simulink model "model_affc"  (R2016b)
settings: Solver=FixedStepDiscrete  StartTime=0.0  StopTime=inf  FixedStep=sampleTime  RelTol=1e-3
PostLoadFcn:
  | model_affc_parameters;
InitFcn:
  | model_affc_parameters;
StartFcn:
  | model_affc_parameters;
values from neighbouring files (symbols this model uses):
  Lb = 0.07    [model_affc_parameters.m]    (also in parameters_sysid.m; parameters_sysid_admittance.m)
  Lf = 0.238    [model_affc_parameters.m]    (also in parameters_sysid.m; parameters_sysid_admittance.m)
  Lu = 0.153    [model_affc_parameters.m]    (also in parameters_sysid.m; parameters_sysid_admittance.m)
  sampleTime = 0.001    [model_affc_parameters.m]    (also in parameters_sysid.m; parameters_sysid_admittance.m)
undefined symbols (not defined in the file or in its folder): FM1
libraries: simulink x14, LibraryFM x14
(part 1 of 2)
settings Model: SimulationMode=external  Creator=niekbeckers  LastModifiedBy=Labuser
settings DataIOCC: LimitDataPoints=on  SaveFormat=Array
settings OptimizationCC: BlockReduction=off  BooleanDataType=off  LocalBlockOutputs=off  LifeSpan=inf
settings DebuggingCC: SaveWithParameterizedLinksMsg=none  UnderspecifiedInitializationDetection=Classic  MergeDetectMultiDrivingBlocksExec=none  SignalResolutionControl=TryResolveAllWithWarning  SFUnexpectedBacktrackingDiag=warning  SFNoUnconditionalDefaultTransitionDiag=warning  SFExecutionAtInitializationDiag=none
settings HardwareCC: ProdBitPerPointer=32  ProdBitPerSizeT=32  ProdBitPerPtrDiffT=32  ProdLargestAtomicFloat=None  ProdIntDivRoundTo=Undefined  ProdEndianess=Unspecified  ProdWordSize=32  ProdHWDeviceType=32-bit Generic  TargetBitPerPointer=64  TargetBitPerSizeT=64  TargetBitPerPtrDiffT=64  TargetLongLongMode=on  TargetIntDivRoundTo=Zero  TargetEndianess=LittleEndian  TargetWordSize=64  TargetHWDeviceType=MATLAB Host  ProdEqTarget=off
settings ModelReferenceCC: PropagateSignalLabelsOutOfModel=off
settings RTWCC: SystemTargetFile=TwinCAT.tlc  GenCodeOnly=on  MakeCommand=make_tct  TemplateMakefile=tct_msbuild.tmf  Description=TwinCAT Target  GenerateReport=on  TargetLang=C++
settings STFCustomTargetCC: CompOptLevelCompliant=on  GeneratePreprocessorConditionals=Disable all  MATLABClassNameForMDSCustomization=Simulink.SoftwareTarget.TargetSpecificTriggerConfigurationBase  SystemTargetFile=TwinCAT.tlc
settings ConfigComp: CovMetricSettings=dw  CovHtmlReporting=on  CovSaveCumulativeToWorkspaceVar=on  CovSaveSingleToWorkspaceVar=on  CovExternalEMLEnable=off  CovSFcnEnable=off

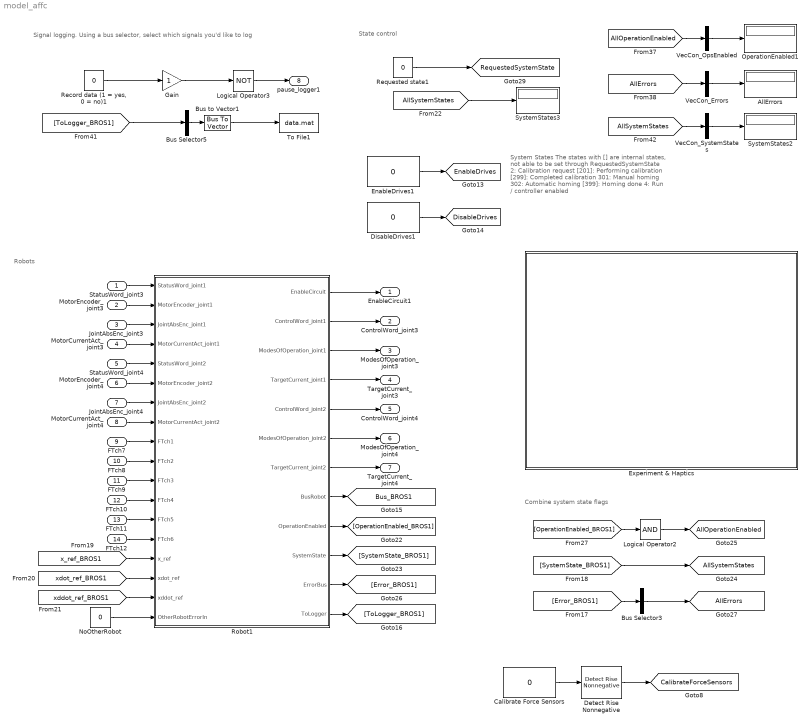
== system model_affc ==
  note: Signal logging.
      | Using a bus selector, select which signals you'd like to log
  note: System States
      | The states with [] are internal states, not able to be set through RequestedSystemState
      | 2: Calibration request
      | [201]: Performing calibration
      | [299]: Completed calibration
      | 301: Manual homing
      | 302: Automatic homing
      | [399]: Homing done
      | 4: Run / controller enabled
  note: State control
  note: Combine system state flags
  note: Robots
  StatusWord_joint3 : Inport  OutDataTypeStr=uint16  PortDimensions=1
  MotorEncoder_joint3 : Inport  Port=2  OutDataTypeStr=int32  PortDimensions=1
  JointAbsEnc_joint3 : Inport  Port=3  OutDataTypeStr=int32  PortDimensions=1
  MotorCurrentAct_joint3 : Inport  Port=4  OutDataTypeStr=int16  PortDimensions=1
  StatusWord_joint4 : Inport  Port=5  OutDataTypeStr=uint16  PortDimensions=1
  MotorEncoder_joint4 : Inport  Port=6  OutDataTypeStr=int32  PortDimensions=1
  JointAbsEnc_joint4 : Inport  Port=7  OutDataTypeStr=int32  PortDimensions=1
  MotorCurrentAct_joint4 : Inport  Port=8  OutDataTypeStr=int16  PortDimensions=1
  FTch7 : Inport  Port=9  OutDataTypeStr=single  PortDimensions=1
  FTch8 : Inport  Port=10  OutDataTypeStr=single  PortDimensions=1
  FTch9 : Inport  Port=11  OutDataTypeStr=single  PortDimensions=1
  FTch10 : Inport  Port=12  OutDataTypeStr=single  PortDimensions=1
  FTch11 : Inport  Port=13  OutDataTypeStr=single  PortDimensions=1
  FTch12 : Inport  Port=14  OutDataTypeStr=single  PortDimensions=1
  AllErrors : Display
  Bus Selector3 : BusSelector  OutputSignals=ErrorCodeLatched  OutputAsBus=on
  Bus Selector5 : BusSelector  OutputSignals=SystemState,qJointSpace.q,qJointSpace.qdot,xOpSpace.x,xOpSpace.xdot,Controller_ToLogger.q_ref,Controller_ToLogger.qdot_ref,Controller_ToLogger.qddot_ref,Controller_ToLogger.p,Controller_ToLogger.tau_affc,BusFTSensor.ForcesOpSpace,ToEtherCAT_ToLogger_Actuator1.DriveError,ToEtherCAT_ToLogger_Actuator2.DriveError  OutputAsBus=on
  Bus to Vector1 : BusToVector
  Calibrate Force Sensors : Constant  Value=0
      settings: OpenFcn=set_param(gcb,'Value','1');tname = ['toggletimer_' gcb];delete(timerfind('name',tname));t = timer('timerfcn', ['set_param(''',gcb,''',''Value'',''0'')'],'executionmode','singleshot','startdelay',1,'name',tname);start(t);
      mask Display: fprintf('PushToTrigger\n%s',get_param(gcb,'value'))
  Detect Rise Nonnegative : simulink/Logic and Bit Operations/Detect Rise Nonnegative  vinit=0  OutDataTypeStr=boolean
  DisableDrives1 : Constant  Value=0
      settings: OpenFcn=set_param(gcb,'Value','1');tname = ['toggletimer_' gcb];delete(timerfind('name',tname));t = timer('timerfcn', ['set_param(''',gcb,''',''Value'',''0'')'],'executionmode','singleshot','startdelay',1,'name',tname);start(t);
      mask Display: fprintf('PushToTrigger\n%s',get_param(gcb,'value'))
  EnableDrives1 : Constant  Value=0
      settings: OpenFcn=set_param(gcb,'Value','1');tname = ['toggletimer_' gcb];delete(timerfind('name',tname));t = timer('timerfcn', ['set_param(''',gcb,''',''Value'',''0'')'],'executionmode','singleshot','startdelay',1,'name',tname);start(t);
      mask Display: fprintf('PushToTrigger\n%s',get_param(gcb,'value'))
  Experiment & Haptics : Subsystem
  Gain : Gain
  Logical Operator2 : Logic  Inputs=1  AllPortsSameDT=off  OutDataTypeStr=boolean
  Logical Operator3 : Logic  Operator=NOT  Inputs=1  AllPortsSameDT=off  OutDataTypeStr=boolean
  NoOtherRobot : Constant  Value=0
  OperationEnabled1 : Display
  "Record data (1 = yes, 0 = no)1" : Constant  Value=0
  Requested state1 : Constant  Value=0
  Robot1 : Subsystem  mask{RobotStruct=FM1}
      mask prompts: RobotStruct "Robot struct (data)"
  SystemStates2 : Display
  SystemStates3 : Display
  To File1 : ToFile  Filename=data.mat  MatrixName=data
  VecCon_Errors : Concatenate  NumInputs=1
  VecCon_OpsEnabled : Concatenate  NumInputs=1
  VecCon_SystemStates : Concatenate  NumInputs=1
  EnableCircuit1 : Outport  OutDataTypeStr=boolean  PortDimensions=1
  ControlWord_joint3 : Outport  Port=2  OutDataTypeStr=uint16  PortDimensions=1
  ModesOfOperation_joint3 : Outport  Port=3  OutDataTypeStr=int8  PortDimensions=1
  TargetCurrent_joint3 : Outport  Port=4  OutDataTypeStr=int16  PortDimensions=1
  ControlWord_joint4 : Outport  Port=5  OutDataTypeStr=uint16  PortDimensions=1
  ModesOfOperation_joint4 : Outport  Port=6  OutDataTypeStr=int8  PortDimensions=1
  TargetCurrent_joint4 : Outport  Port=7  OutDataTypeStr=int16  PortDimensions=1
  pause_logger1 : Outport  Port=8  OutDataTypeStr=boolean  PortDimensions=1
  tag scope: AllErrors=global, AllOperationEnabled=global, AllSystemStates=global, Bus_BROS1=global, CalibrateForceSensors=global, DisableDrives=global, EnableDrives=global, RequestedSystemState=global
  wires:
  DisableDrives1/1 -> [DisableDrives]
  EnableDrives1/1 -> [EnableDrives]
  Robot1/9(OperationEnabled) -> [OperationEnabled_BROS1]
  [AllOperationEnabled] -> VecCon_OpsEnabled/1
  Robot1/10(SystemState) -> [SystemState_BROS1]
  [SystemState_BROS1] -> [AllSystemStates]
  Logical Operator2/1 -> [AllOperationEnabled]
  [OperationEnabled_BROS1] -> Logical Operator2/1
  Robot1/11(ErrorBus) -> [Error_BROS1]
  [Error_BROS1] -> Bus Selector3/1
  [AllErrors] -> VecCon_Errors/1
  [x_ref_BROS1] -> Robot1/15(x_ref)
  [xdot_ref_BROS1] -> Robot1/16(xdot_ref)
  [xddot_ref_BROS1] -> Robot1/17(xddot_ref)
  Requested state1/1 -> [RequestedSystemState]
  Robot1/8(BusRobot) -> [Bus_BROS1]
  StatusWord_joint3/1 -> Robot1/1(StatusWord_joint1)
  MotorEncoder_joint3/1 -> Robot1/2(MotorEncoder_joint1)
  JointAbsEnc_joint3/1 -> Robot1/3(JointAbsEnc_joint1)
  MotorCurrentAct_joint3/1 -> Robot1/4(MotorCurrentAct_joint1)
  StatusWord_joint4/1 -> Robot1/5(StatusWord_joint2)
  MotorEncoder_joint4/1 -> Robot1/6(MotorEncoder_joint2)
  JointAbsEnc_joint4/1 -> Robot1/7(JointAbsEnc_joint2)
  MotorCurrentAct_joint4/1 -> Robot1/8(MotorCurrentAct_joint2)
  FTch7/1 -> Robot1/9(FTch1)
  FTch8/1 -> Robot1/10(FTch2)
  FTch9/1 -> Robot1/11(FTch3)
  FTch10/1 -> Robot1/12(FTch4)
  FTch11/1 -> Robot1/13(FTch5)
  FTch12/1 -> Robot1/14(FTch6)
  Robot1/2(ControlWord_joint1) -> ControlWord_joint3/1
  Robot1/3(ModesOfOperation_joint1) -> ModesOfOperation_joint3/1
  Robot1/4(TargetCurrent_joint1) -> TargetCurrent_joint3/1
  Robot1/7(TargetCurrent_joint2) -> TargetCurrent_joint4/1
  Robot1/6(ModesOfOperation_joint2) -> ModesOfOperation_joint4/1
  Robot1/5(ControlWord_joint2) -> ControlWord_joint4/1
  Robot1/12(ToLogger) -> [ToLogger_BROS1]
  [ToLogger_BROS1] -> Bus Selector5/1
  [AllSystemStates] -> SystemStates3/1
  Logical Operator3/1 -> pause_logger1/1
  Bus Selector5/1 -> Bus to Vector1/1
  Bus Selector3/1 -> [AllErrors]
  Bus to Vector1/1 -> To File1/1
  Robot1/1(EnableCircuit) -> EnableCircuit1/1
  NoOtherRobot/1 -> Robot1/18(OtherRobotErrorIn)
  VecCon_Errors/1 -> AllErrors/1
  [AllSystemStates] -> VecCon_SystemStates/1
  VecCon_SystemStates/1 -> SystemStates2/1
  VecCon_OpsEnabled/1 -> OperationEnabled1/1
  "Record data (1 = yes, 0 = no)1"/1 -> Gain/1
  Calibrate Force Sensors/1 -> Detect Rise Nonnegative/1
  Detect Rise Nonnegative/1 -> [CalibrateForceSensors]
  Gain/1 -> Logical Operator3/1

== system model_affc/Experiment & Haptics ==
  note: Only run trajectory if all systems are in state 4 (run)
  Add : Sum
  "Check state " : simulink/Logic and Bit Operations/Compare To Constant  relop===  const=4  OutDataTypeStr=boolean
  Constant : Constant  Value=FM1.HomeLocationOpSpace
  Hypotrochoid trajectory for AFFC : Subsystem
  Logical Operator : Logic  Inputs=1  AllPortsSameDT=off  OutDataTypeStr=boolean
  Terminator1 : Terminator
  tag scope: x_ref_BROS1=global, xddot_ref_BROS1=global, xdot_ref_BROS1=global
  wires:
  [Bus_BROS1] -> Terminator1/1
  Constant/1 -> Add/1
  Hypotrochoid trajectory for AFFC/1(dx_ref) -> Add/2
  Add/1 -> [x_ref_BROS1]
  Hypotrochoid trajectory for AFFC/2(dxdot_ref) -> [xdot_ref_BROS1]
  Hypotrochoid trajectory for AFFC/3(dxddot_ref) -> [xddot_ref_BROS1]
  [AllSystemStates] -> "Check state "/1
  "Check state "/1 -> Logical Operator/1
  Logical Operator/1 -> Hypotrochoid trajectory for AFFC/Enable

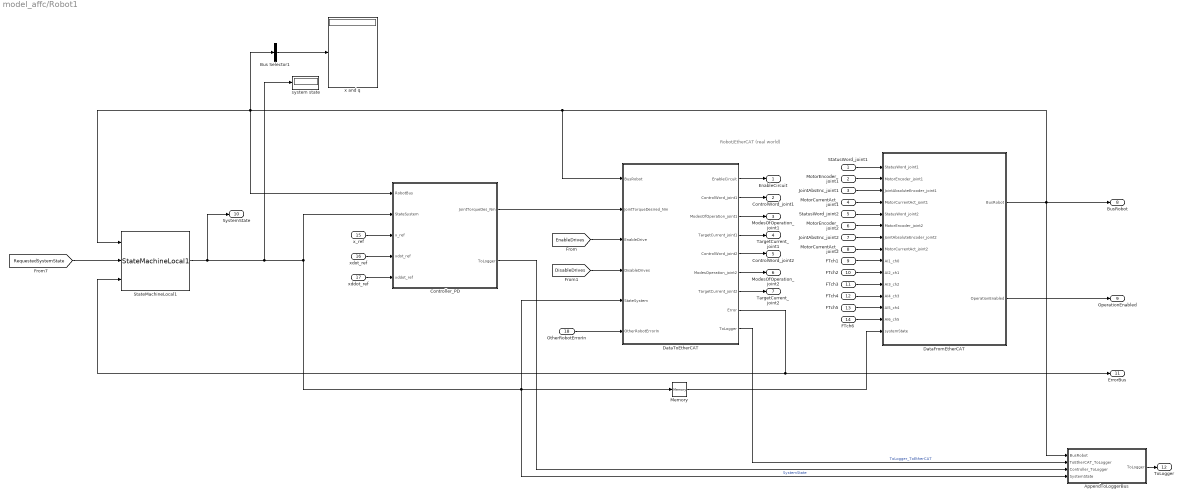
== system model_affc/Robot1 ==
  note: Robot/EtherCAT (real world)
  StatusWord_joint1 : Inport
  MotorEncoder_joint1 : Inport  Port=2
  JointAbsEnc_joint1 : Inport  Port=3
  MotorCurrentAct_joint1 : Inport  Port=4
  StatusWord_joint2 : Inport  Port=5
  MotorEncoder_joint2 : Inport  Port=6
  JointAbsEnc_joint2 : Inport  Port=7
  MotorCurrentAct_joint2 : Inport  Port=8
  FTch1 : Inport  Port=9
  FTch2 : Inport  Port=10
  FTch3 : Inport  Port=11
  FTch4 : Inport  Port=12
  FTch5 : Inport  Port=13
  FTch6 : Inport  Port=14
  x_ref : Inport  Port=15
  xdot_ref : Inport  Port=16
  xddot_ref : Inport  Port=17
  OtherRobotErrorIn : Inport  Port=18
  AppendToLoggerBus : Subsystem
  Bus Selector1 : BusSelector  OutputSignals=qJointSpace.q,qJointSpace.qdot,xOpSpace.x,BusActuators.BusActuator1.JointPosition_AbsEnc_rad,BusActuators.BusActuator2.JointPosition_AbsEnc_rad  OutputAsBus=on
  Controller_PD : Subsystem
  DataFromEtherCAT : Subsystem
  DataToEtherCAT : Subsystem
  Memory : Memory
  StateMachineLocal1 : LibraryFM/StateMachineLocal1
  system state : Display
  x and q : Display
  EnableCircuit : Outport
  ControlWord_joint1 : Outport  Port=2
  ModesOfOperation_joint1 : Outport  Port=3
  TargetCurrent_joint1 : Outport  Port=4
  ControlWord_joint2 : Outport  Port=5
  ModesOfOperation_joint2 : Outport  Port=6
  TargetCurrent_joint2 : Outport  Port=7
  BusRobot : Outport  Port=8
  OperationEnabled : Outport  Port=9
  SystemState : Outport  Port=10
  ErrorBus : Outport  Port=11
  ToLogger : Outport  Port=12
  wires:
  xddot_ref/1 -> Controller_PD/5(xddot_ref)
  xdot_ref/1 -> Controller_PD/4(xdot_ref)
  x_ref/1 -> Controller_PD/3(x_ref)
  DataToEtherCAT/7(TargetCurrent_joint2) -> TargetCurrent_joint2/1
  FTch2/1 -> DataFromEtherCAT/10(AI2_ch1)
  MotorCurrentAct_joint1/1 -> DataFromEtherCAT/4(MotorCurrentAct_joint1)
  MotorEncoder_joint2/1 -> DataFromEtherCAT/6(MotorEncoder_joint2)
  JointAbsEnc_joint1/1 -> DataFromEtherCAT/3(JointAbsoluteEncoder_joint1)
  DataToEtherCAT/3(ModesOfOperation_joint1) -> ModesOfOperation_joint1/1
  DataToEtherCAT/1(EnableCircuit) -> EnableCircuit/1
  FTch1/1 -> DataFromEtherCAT/9(AI1_ch0)
  StateMachineLocal1/1 -> system state/1, Controller_PD/2(StateSystem), DataToEtherCAT/5(StateSystem), Memory/1, AppendToLoggerBus/4(SystemState), SystemState/1  "SystemState"
  DataToEtherCAT/2(ControlWord_joint1) -> ControlWord_joint1/1
  DataToEtherCAT/8(Error) -> StateMachineLocal1/3, ErrorBus/1
  DataFromEtherCAT/1(BusRobot) -> AppendToLoggerBus/1(BusRobot), Controller_PD/1(RobotBus), StateMachineLocal1/1, Bus Selector1/1, DataToEtherCAT/1(BusRobot), BusRobot/1
  [RequestedSystemState] -> StateMachineLocal1/2
  Controller_PD/1(JointTorqueDes_Nm) -> DataToEtherCAT/2(JointTorqueDesired_Nm)
  [DisableDrives] -> DataToEtherCAT/4(DisableDrives)
  [EnableDrives] -> DataToEtherCAT/3(EnableDrive)
  MotorCurrentAct_joint2/1 -> DataFromEtherCAT/8(MotorCurrentAct_joint2)
  DataToEtherCAT/4(TargetCurrent_joint1) -> TargetCurrent_joint1/1
  FTch5/1 -> DataFromEtherCAT/13(AI5_ch4)
  JointAbsEnc_joint2/1 -> DataFromEtherCAT/7("JointAbsoluteEncoder_joint2 ")
  MotorEncoder_joint1/1 -> DataFromEtherCAT/2(MotorEncoder_joint1)
  DataToEtherCAT/5(ControlWord_joint2) -> ControlWord_joint2/1
  DataToEtherCAT/6(ModesOperation_joint2) -> ModesOfOperation_joint2/1
  StatusWord_joint1/1 -> DataFromEtherCAT/1(StatusWord_joint1)
  StatusWord_joint2/1 -> DataFromEtherCAT/5(StatusWord_joint2)
  FTch6/1 -> DataFromEtherCAT/14(AI6_ch5)
  FTch4/1 -> DataFromEtherCAT/12(AI4_ch3)
  FTch3/1 -> DataFromEtherCAT/11(AI3_ch2)
  DataFromEtherCAT/2(OperationEnabled) -> OperationEnabled/1
  Bus Selector1/1 -> x and q/1
  Controller_PD/2(ToLogger) -> AppendToLoggerBus/3(Controller_ToLogger)
  DataToEtherCAT/9(ToLogger) -> AppendToLoggerBus/2(ToEtherCAT_ToLogger)  "ToLogger_ToEtherCAT"
  AppendToLoggerBus/1(ToLogger) -> ToLogger/1
  Memory/1 -> DataFromEtherCAT/15(systemState)
  OtherRobotErrorIn/1 -> DataToEtherCAT/6(OtherRobotErrorIn)

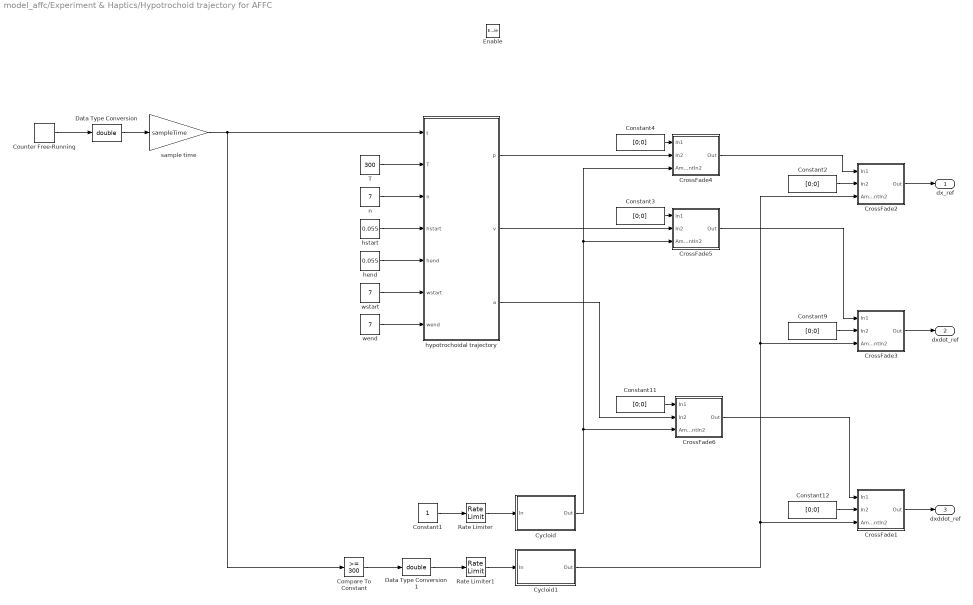
== system model_affc/Experiment & Haptics/Hypotrochoid trajectory for AFFC ==
  Enable : EnablePort  StatesWhenEnabling=reset
  Compare To Constant : simulink/Logic and Bit Operations/Compare To Constant  relop=>=  const=300  OutDataTypeStr=boolean
  Constant1 : Constant
  Constant{2..4,9,11..12} (6 alike) : Constant  Value=[0;0]
  Counter Free-Running : simulink/Sources/Counter Free-Running  NumBits=32  tsamp=-1
  CrossFade1 : Subsystem  AncestorBlock=VariousBlocksLibrary/Various/CrossFade
  CrossFade2 : Subsystem  AncestorBlock=VariousBlocksLibrary/Various/CrossFade
  CrossFade3 : Subsystem  AncestorBlock=VariousBlocksLibrary/Various/CrossFade
  CrossFade4 : Subsystem
  CrossFade5 : Subsystem  AncestorBlock=VariousBlocksLibrary/Various/CrossFade
  CrossFade6 : Subsystem  AncestorBlock=VariousBlocksLibrary/Various/CrossFade
  Cycloid : Subsystem  AncestorBlock=VariousBlocksLibrary/Various/Cycloid
  Cycloid1 : Subsystem  AncestorBlock=VariousBlocksLibrary/Various/Cycloid
  Data Type Conversion : DataTypeConversion  OutDataTypeStr=double
  Data Type Conversion1 : DataTypeConversion  OutDataTypeStr=double
  Rate Limiter : RateLimiter  RisingSlewLimit=0.25  FallingSlewLimit=-0.15  SampleTimeMode=inherited
  Rate Limiter1 : RateLimiter  RisingSlewLimit=0.2  FallingSlewLimit=-0.2  SampleTimeMode=inherited
  T : Constant  Value=300
  hend : Constant  Value=0.055
  hstart : Constant  Value=0.055
  hypotrochoidal trajectory : MATLAB Function  TreatAsAtomicUnit=on
  n : Constant  Value=7
  sample time : Gain  Gain=sampleTime
  wend : Constant  Value=7
  wstart : Constant  Value=7
  dx_ref : Outport  InitialOutput=[0;0]
  dxdot_ref : Outport  Port=2  InitialOutput=[0;0]
  dxddot_ref : Outport  Port=3  InitialOutput=[0;0]
  wires:
  Data Type Conversion1/1 -> Rate Limiter1/1
  hypotrochoidal trajectory/1(p) -> CrossFade4/2(In2)
  CrossFade1/1(Out) -> dxddot_ref/1
  Constant11/1 -> CrossFade6/1(In1)
  Constant12/1 -> CrossFade1/2(In2)
  CrossFade6/1(Out) -> CrossFade1/1(In1)
  Constant9/1 -> CrossFade3/2(In2)
  CrossFade5/1(Out) -> CrossFade3/1(In1)
  CrossFade3/1(Out) -> dxdot_ref/1
  Cycloid1/1(Out) -> CrossFade1/3(AmountIn2), CrossFade2/3(AmountIn2), CrossFade3/3(AmountIn2)
  Rate Limiter1/1 -> Cycloid1/1(In)
  Compare To Constant/1 -> Data Type Conversion1/1
  CrossFade4/1(Out) -> CrossFade2/1(In1)
  CrossFade2/1(Out) -> dx_ref/1
  Rate Limiter/1 -> Cycloid/1(In)
  Constant1/1 -> Rate Limiter/1
  Cycloid/1(Out) -> CrossFade6/3(AmountIn2), CrossFade5/3(AmountIn2), CrossFade4/3(AmountIn2)
  hypotrochoidal trajectory/2(v) -> CrossFade5/2(In2)
  hypotrochoidal trajectory/3(a) -> CrossFade6/2(In2)
  sample time/1 -> Compare To Constant/1, hypotrochoidal trajectory/1(t)
  Constant2/1 -> CrossFade2/2(In2)
  Data Type Conversion/1 -> sample time/1
  wstart/1 -> hypotrochoidal trajectory/6(wstart)
  wend/1 -> hypotrochoidal trajectory/7(wend)
  hstart/1 -> hypotrochoidal trajectory/4(hstart)
  hend/1 -> hypotrochoidal trajectory/5(hend)
  n/1 -> hypotrochoidal trajectory/3(n)
  T/1 -> hypotrochoidal trajectory/2(T)
  Counter Free-Running/1 -> Data Type Conversion/1
  Constant3/1 -> CrossFade5/1(In1)
  Constant4/1 -> CrossFade4/1(In1)

== system model_affc/Robot1/AppendToLoggerBus ==
  BusRobot : Inport
  ToEtherCAT_ToLogger : Inport  Port=2
  Controller_ToLogger : Inport  Port=3
  SystemState : Inport  Port=4
  Bus Creator : BusCreator  Inputs=8
  Bus Selector : BusSelector  OutputSignals=xOpSpace,qJointSpace,BusFTSensor,BusActuators
  Bus Selector1 : BusSelector  OutputSignals=ToEtherCAT_ToLogger_Actuator1,ToEtherCAT_ToLogger_Actuator2
  ToLogger : Outport
  wires:
  Bus Creator/1 -> ToLogger/1  "LoggerBus"
  Bus Selector/4 -> Bus Creator/4  "<BusActuators>"
  Bus Selector/1 -> Bus Creator/1  "<xOpSpace>"
  Bus Selector/3 -> Bus Creator/3  "<BusFTSensor>"
  Bus Selector/2 -> Bus Creator/2  "<qJointSpace>"
  BusRobot/1 -> Bus Selector/1
  ToEtherCAT_ToLogger/1 -> Bus Selector1/1
  Bus Selector1/1 -> Bus Creator/5  "<ToEtherCAT_ToLogger_Actuator1>"
  Bus Selector1/2 -> Bus Creator/6  "<ToEtherCAT_ToLogger_Actuator2>"
  Controller_ToLogger/1 -> Bus Creator/7
  SystemState/1 -> Bus Creator/8  "SystemState"

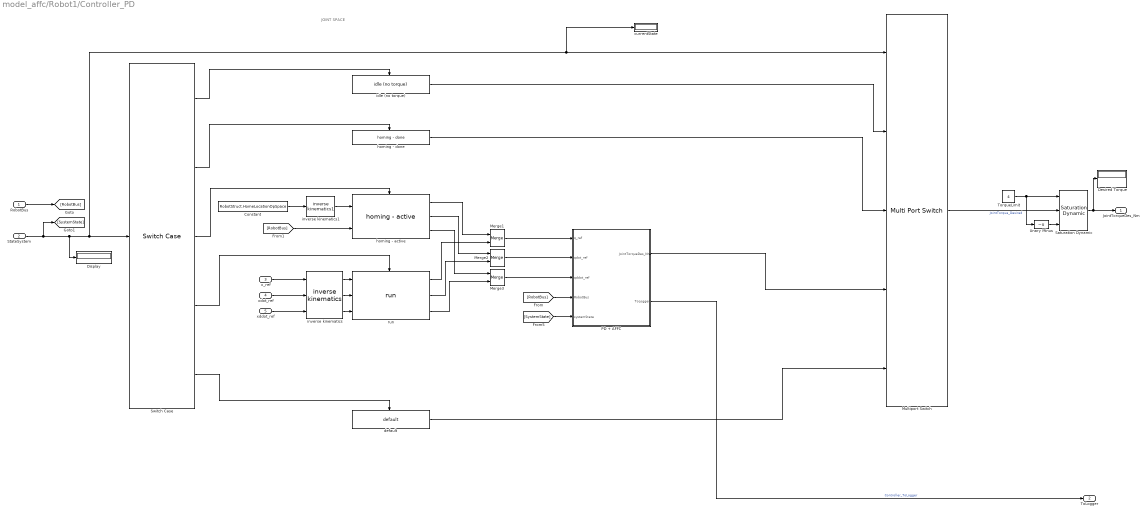
== system model_affc/Robot1/Controller_PD ==
  note: JOINT SPACE
  RobotBus : Inport
  StateSystem : Inport  Port=2
  x_ref : Inport  Port=3
  xdot_ref : Inport  Port=4
  xddot_ref : Inport  Port=5
  Constant : Constant  Value=RobotStruct.HomeLocationOpSpace
  Desired Torque : Display
  Display : Display
  Merge1 : Merge  InitialOutput=[0;0]
  Merge2 : Merge  InitialOutput=[0;0]
  Merge3 : Merge  InitialOutput=[0;0]
  Multiport Switch : MultiPortSwitch  DataPortOrder=Specify indices  Inputs=4  DataPortIndices={[0,1,2,201,299,301],[399],[302,4]}  DataPortForDefault=Additional data port
  PD + AFFC : Subsystem  AncestorBlock=LibraryFM/PD + AFFC
  Saturation Dynamic : simulink/Discontinuities/Saturation Dynamic  OutMin=[]  OutMax=[]  OutDataTypeStr=Inherit: Same as second input  OutDataType=fixdt(1, 16)  OutScaling=2^-10  DoSatur=off
  Switch Case : SwitchCase  CaseConditions={[0,1,2,201,299,301],[399],[302],[4]}
  TorqueLimit : Constant  Value=4
  Unary Minus : UnaryMinus
  currentState : Display
  default : LibraryFM/Controller_AFFC/default
  homing - active : LibraryFM/Controller_AFFC/homing - active
      link override CrossFade: SourceBlock=LibraryFM/Utilities/CrossFade
      link override Cycloid: SourceBlock=LibraryFM/Utilities/Cycloid
  homing - done : LibraryFM/Controller_AFFC/homing - done
  idle (no torque) : LibraryFM/Controller_AFFC/idle (no torque)
  inverse kinematics : LibraryFM/Controller_AFFC/inverse kinematics
  inverse kinematics1 : LibraryFM/Controller_AFFC/inverse kinematics1
  run : LibraryFM/Controller_AFFC/run
  JointTorqueDes_Nm : Outport
  ToLogger : Outport  Port=2
  wires:
  Saturation Dynamic/1 -> Desired Torque/1, JointTorqueDes_Nm/1
  TorqueLimit/1 -> Unary Minus/1, Saturation Dynamic/1
  Unary Minus/1 -> Saturation Dynamic/3
  xdot_ref/1 -> inverse kinematics/2
  xddot_ref/1 -> inverse kinematics/3
  x_ref/1 -> inverse kinematics/1
  [SystemState] -> PD + AFFC/5(systemState)
  inverse kinematics/3 -> run/3
  inverse kinematics/2 -> run/2
  inverse kinematics/1 -> run/1
  Constant/1 -> inverse kinematics1/1
  [RobotBus] -> homing - active/2
  [RobotBus] -> PD + AFFC/4(RobotBus)
  RobotBus/1 -> [RobotBus]
  PD + AFFC/1(JointTorqueDes_Nm) -> Multiport Switch/4
  Merge3/1 -> PD + AFFC/3(qddot_ref)
  Merge2/1 -> PD + AFFC/2(qdot_ref)
  Merge1/1 -> PD + AFFC/1(q_ref)
  homing - done/1 -> Multiport Switch/3
  idle (no torque)/1 -> Multiport Switch/2
  Switch Case/2 -> homing - done/Action
  Switch Case/3 -> homing - active/Action
  Switch Case/1 -> idle (no torque)/Action
  default/1 -> Multiport Switch/5
  Switch Case/5 -> default/Action
  Switch Case/4 -> run/Action
  homing - active/1 -> Merge1/1
  run/1 -> Merge1/2
  StateSystem/1 -> Display/1, Multiport Switch/1, currentState/1, Switch Case/1, [SystemState]
  run/2 -> Merge2/2
  run/3 -> Merge3/2
  homing - active/2 -> Merge2/1
  homing - active/3 -> Merge3/1
  Multiport Switch/1 -> Saturation Dynamic/2  "JointTorque_Desired"
  inverse kinematics1/1 -> homing - active/1
  PD + AFFC/2(ToLogger) -> ToLogger/1  "Controller_ToLogger"

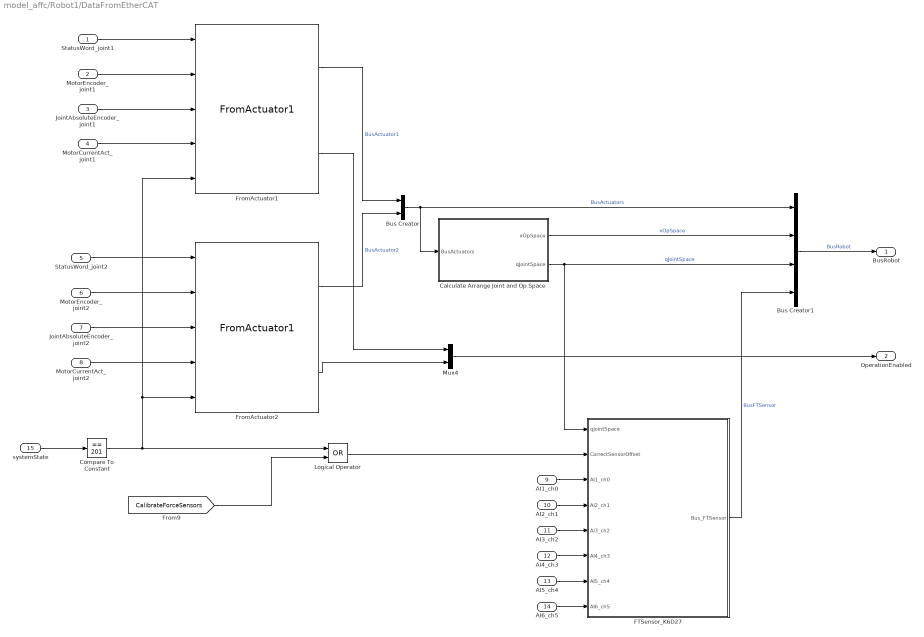
== system model_affc/Robot1/DataFromEtherCAT ==
  StatusWord_joint1 : Inport
  MotorEncoder_joint1 : Inport  Port=2
  JointAbsoluteEncoder_joint1 : Inport  Port=3
  MotorCurrentAct_joint1 : Inport  Port=4
  StatusWord_joint2 : Inport  Port=5
  MotorEncoder_joint2 : Inport  Port=6
  "JointAbsoluteEncoder_joint2 " : Inport  Port=7
  MotorCurrentAct_joint2 : Inport  Port=8
  AI1_ch0 : Inport  Port=9
  AI2_ch1 : Inport  Port=10
  AI3_ch2 : Inport  Port=11
  AI4_ch3 : Inport  Port=12
  AI5_ch4 : Inport  Port=13
  AI6_ch5 : Inport  Port=14
  systemState : Inport  Port=15
  Bus Creator : BusCreator  Inputs=2
  Bus Creator1 : BusCreator  Inputs=4
  Calculate Arrange Joint and Op Space : Subsystem
  Compare To Constant : simulink/Logic and Bit Operations/Compare To Constant  relop===  const=201  OutDataTypeStr=boolean
  FTSensor_K6D27 : Subsystem  mask{FTSensorStruct=RobotStruct.FTSensor}
      mask prompts: FTSensorStruct "Struct for force torque sensor"
  FromActuator1 : LibraryFM/FromActuator1  ActuatorStruct=RobotStruct.Actuator1
  FromActuator2 : LibraryFM/FromActuator1  ActuatorStruct=RobotStruct.Actuator2
  Logical Operator : Logic  Operator=OR  AllPortsSameDT=off  OutDataTypeStr=boolean
  Mux4 : Mux  Inputs=2
  BusRobot : Outport
  OperationEnabled : Outport  Port=2
  wires:
  FTSensor_K6D27/1(Bus_FTSensor) -> Bus Creator1/4  "BusFTSensor"
  FromActuator1/1 -> Bus Creator/1  "BusActuator1"
  FromActuator2/1 -> Bus Creator/2  "BusActuator2"
  FromActuator1/2 -> Mux4/1
  Mux4/1 -> OperationEnabled/1
  FromActuator2/2 -> Mux4/2
  MotorEncoder_joint1/1 -> FromActuator1/2
  StatusWord_joint1/1 -> FromActuator1/1
  JointAbsoluteEncoder_joint1/1 -> FromActuator1/3
  MotorCurrentAct_joint1/1 -> FromActuator1/4
  MotorEncoder_joint2/1 -> FromActuator2/2
  StatusWord_joint2/1 -> FromActuator2/1
  "JointAbsoluteEncoder_joint2 "/1 -> FromActuator2/3
  MotorCurrentAct_joint2/1 -> FromActuator2/4
  Bus Creator/1 -> Calculate Arrange Joint and Op Space/1(BusActuators), Bus Creator1/1  "BusActuators"
  Bus Creator1/1 -> BusRobot/1  "BusRobot"
  Calculate Arrange Joint and Op Space/2(qJointSpace) -> FTSensor_K6D27/1(qJointSpace), Bus Creator1/3  "qJointSpace"
  systemState/1 -> Compare To Constant/1
  AI1_ch0/1 -> FTSensor_K6D27/3(AI1_ch0)
  AI2_ch1/1 -> FTSensor_K6D27/4(AI2_ch1)
  AI3_ch2/1 -> FTSensor_K6D27/5(AI3_ch2)
  AI4_ch3/1 -> FTSensor_K6D27/6(AI4_ch3)
  AI5_ch4/1 -> FTSensor_K6D27/7(AI5_ch4)
  AI6_ch5/1 -> FTSensor_K6D27/8(AI6_ch5)
  Compare To Constant/1 -> FromActuator1/5, FromActuator2/5, Logical Operator/1
  Calculate Arrange Joint and Op Space/1(xOpSpace) -> Bus Creator1/2  "xOpSpace"
  [CalibrateForceSensors] -> Logical Operator/2
  Logical Operator/1 -> FTSensor_K6D27/2(CorrectSensorOffset)

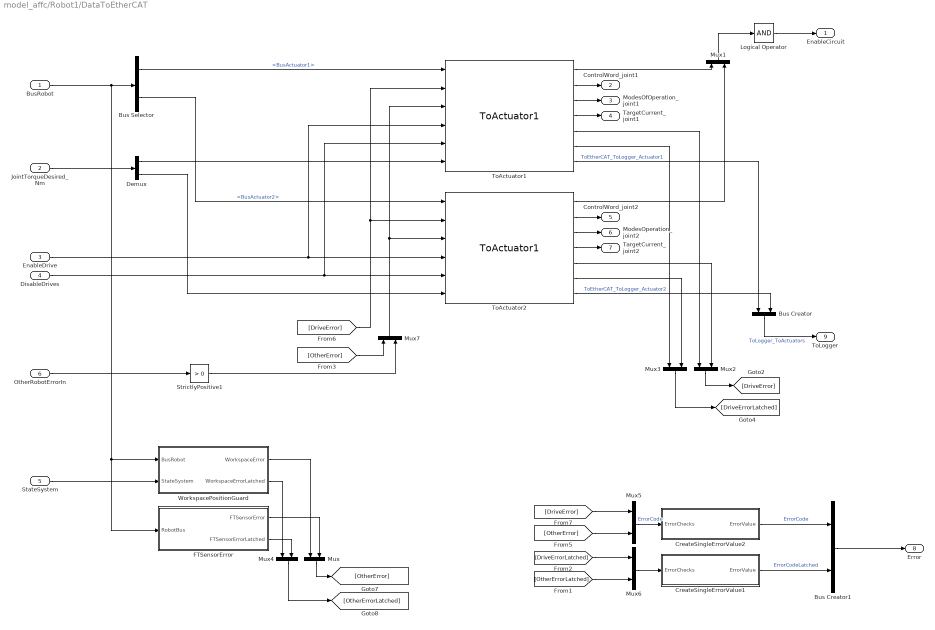
== system model_affc/Robot1/DataToEtherCAT ==
  BusRobot : Inport
  JointTorqueDesired_Nm : Inport  Port=2
  EnableDrive : Inport  Port=3
  DisableDrives : Inport  Port=4
  StateSystem : Inport  Port=5
  OtherRobotErrorIn : Inport  Port=6
  Bus Creator : BusCreator  Inputs=2
  Bus Creator1 : BusCreator  Inputs=2
  Bus Selector : BusSelector  OutputSignals=BusActuators.BusActuator1,BusActuators.BusActuator2
  CreateSingleErrorValue1 : Subsystem
  CreateSingleErrorValue2 : Subsystem
  Demux : Demux  Outputs=2
  FTSensorError : Subsystem
  Logical Operator : Logic  Inputs=1  AllPortsSameDT=off  OutDataTypeStr=boolean
  Mux{,1..7} (8 alike) : Mux  Inputs=2
  StrictlyPositive1 : simulink/Logic and Bit Operations/Compare To Zero  relop=>  OutDataTypeStr=boolean
  ToActuator1 : LibraryFM/ToActuator1  ActuatorStruct=RobotStruct.Actuator1
      link override DriveEnableLogic/8_JointVelocityGuard/Constant: Value=3*pi
  ToActuator2 : LibraryFM/ToActuator1  ActuatorStruct=RobotStruct.Actuator2
      link override DriveEnableLogic/8_JointVelocityGuard/Constant: Value=3*pi
  WorkspacePositionGuard : Subsystem
  EnableCircuit : Outport  OutDataTypeStr=boolean
  ControlWord_joint1 : Outport  Port=2  OutDataTypeStr=uint16
  ModesOfOperation_joint1 : Outport  Port=3  OutDataTypeStr=int8
  TargetCurrent_joint1 : Outport  Port=4  OutDataTypeStr=int16
  ControlWord_joint2 : Outport  Port=5  OutDataTypeStr=uint16
  ModesOperation_joint2 : Outport  Port=6  OutDataTypeStr=int8
  TargetCurrent_joint2 : Outport  Port=7  OutDataTypeStr=int16
  Error : Outport  Port=8
  ToLogger : Outport  Port=9
  wires:
  Bus Creator/1 -> ToLogger/1  "ToLogger_ToActuators"
  ToActuator2/7 -> Bus Creator/2  "ToEtherCAT_ToLogger_Actuator2"
  ToActuator1/7 -> Bus Creator/1  "ToEtherCAT_ToLogger_Actuator1"
  ToActuator1/5 -> Mux2/1
  ToActuator2/5 -> Mux2/2
  Mux2/1 -> [DriveError]
  ToActuator1/6 -> Mux3/1
  ToActuator2/6 -> Mux3/2
  [DriveError] -> ToActuator1/2, ToActuator2/2
  Mux1/1 -> Logical Operator/1
  ToActuator1/1 -> Mux1/1
  ToActuator2/1 -> Mux1/2
  ToActuator1/2 -> ControlWord_joint1/1
  ToActuator1/3 -> ModesOfOperation_joint1/1
  ToActuator2/2 -> ControlWord_joint2/1
  ToActuator1/4 -> TargetCurrent_joint1/1
  ToActuator2/4 -> TargetCurrent_joint2/1
  ToActuator2/3 -> ModesOperation_joint2/1
  Logical Operator/1 -> EnableCircuit/1
  Demux/2 -> ToActuator2/6
  JointTorqueDesired_Nm/1 -> Demux/1
  Demux/1 -> ToActuator1/6
  BusRobot/1 -> WorkspacePositionGuard/1(BusRobot), FTSensorError/1(RobotBus), Bus Selector/1
  Bus Selector/2 -> ToActuator2/1  "<BusActuator2>"
  Bus Selector/1 -> ToActuator1/1  "<BusActuator1>"
  DisableDrives/1 -> ToActuator1/5, ToActuator2/5
  EnableDrive/1 -> ToActuator1/4, ToActuator2/4
  Mux3/1 -> [DriveErrorLatched]
  StateSystem/1 -> WorkspacePositionGuard/2(StateSystem)
  FTSensorError/1(FTSensorError) -> Mux/2
  FTSensorError/2(FTSensorErrorLatched) -> Mux4/2
  WorkspacePositionGuard/1(WorkspaceError) -> Mux/1
  WorkspacePositionGuard/2(WorkspaceErrorLatched) -> Mux4/1
  Mux/1 -> [OtherError]
  Mux4/1 -> [OtherErrorLatched]
  [DriveError] -> Mux5/1
  [OtherError] -> Mux5/2
  CreateSingleErrorValue1/1(ErrorValue) -> Bus Creator1/2  "ErrorCodeLatched"
  [DriveErrorLatched] -> Mux6/1
  [OtherErrorLatched] -> Mux6/2
  Mux6/1 -> CreateSingleErrorValue1/1(ErrorChecks)
  Mux5/1 -> CreateSingleErrorValue2/1(ErrorChecks)  "ErrorCode"
  Bus Creator1/1 -> Error/1
  CreateSingleErrorValue2/1(ErrorValue) -> Bus Creator1/1  "ErrorCode"
  [OtherError] -> Mux7/1
  Mux7/1 -> ToActuator2/3, ToActuator1/3
  OtherRobotErrorIn/1 -> StrictlyPositive1/1
  StrictlyPositive1/1 -> Mux7/2

== system model_affc/Experiment & Haptics/Hypotrochoid trajectory for AFFC/CrossFade1 ==
  In1 : Inport
  In2 : Inport  Port=2
  AmountIn2 : Inport  Port=3
  Add : Sum  Inputs=+-
  Add1 : Sum
  One : Constant
  Product : Product  RndMeth=Zero
  Product1 : Product  RndMeth=Zero
  Saturation : Saturate  UpperLimit=1  LowerLimit=0
  Out : Outport
  wires:
  In1/1 -> Product1/1
  AmountIn2/1 -> Saturation/1
  One/1 -> Add/1
  Saturation/1 -> Product/2, Add/2
  Add/1 -> Product1/2
  Product/1 -> Add1/2
  Product1/1 -> Add1/1
  In2/1 -> Product/1
  Add1/1 -> Out/1

== system model_affc/Experiment & Haptics/Hypotrochoid trajectory for AFFC/CrossFade2 ==
  In1 : Inport
  In2 : Inport  Port=2
  AmountIn2 : Inport  Port=3
  Add : Sum  Inputs=+-
  Add1 : Sum
  One : Constant
  Product : Product  RndMeth=Zero
  Product1 : Product  RndMeth=Zero
  Saturation : Saturate  UpperLimit=1  LowerLimit=0
  Out : Outport
  wires:
  In1/1 -> Product1/1
  AmountIn2/1 -> Saturation/1
  One/1 -> Add/1
  Saturation/1 -> Product/2, Add/2
  Add/1 -> Product1/2
  Product/1 -> Add1/2
  Product1/1 -> Add1/1
  In2/1 -> Product/1
  Add1/1 -> Out/1

== system model_affc/Experiment & Haptics/Hypotrochoid trajectory for AFFC/CrossFade3 ==
  In1 : Inport
  In2 : Inport  Port=2
  AmountIn2 : Inport  Port=3
  Add : Sum  Inputs=+-
  Add1 : Sum
  One : Constant
  Product : Product  RndMeth=Zero
  Product1 : Product  RndMeth=Zero
  Saturation : Saturate  UpperLimit=1  LowerLimit=0
  Out : Outport
  wires:
  In1/1 -> Product1/1
  AmountIn2/1 -> Saturation/1
  One/1 -> Add/1
  Saturation/1 -> Product/2, Add/2
  Add/1 -> Product1/2
  Product/1 -> Add1/2
  Product1/1 -> Add1/1
  In2/1 -> Product/1
  Add1/1 -> Out/1

== system model_affc/Experiment & Haptics/Hypotrochoid trajectory for AFFC/CrossFade4 ==
  In1 : Inport
  In2 : Inport  Port=2
  AmountIn2 : Inport  Port=3
  Add : Sum  Inputs=+-
  Add1 : Sum
  One : Constant
  Product : Product  RndMeth=Zero
  Product1 : Product  RndMeth=Zero
  Saturation : Saturate  UpperLimit=1  LowerLimit=0
  Out : Outport
  wires:
  In1/1 -> Product1/1
  AmountIn2/1 -> Saturation/1
  One/1 -> Add/1
  Saturation/1 -> Product/2, Add/2
  Add/1 -> Product1/2
  Product/1 -> Add1/2
  Product1/1 -> Add1/1
  In2/1 -> Product/1
  Add1/1 -> Out/1

== system model_affc/Experiment & Haptics/Hypotrochoid trajectory for AFFC/CrossFade5 ==
  In1 : Inport
  In2 : Inport  Port=2
  AmountIn2 : Inport  Port=3
  Add : Sum  Inputs=+-
  Add1 : Sum
  One : Constant
  Product : Product  RndMeth=Zero
  Product1 : Product  RndMeth=Zero
  Saturation : Saturate  UpperLimit=1  LowerLimit=0
  Out : Outport
  wires:
  In1/1 -> Product1/1
  AmountIn2/1 -> Saturation/1
  One/1 -> Add/1
  Saturation/1 -> Product/2, Add/2
  Add/1 -> Product1/2
  Product/1 -> Add1/2
  Product1/1 -> Add1/1
  In2/1 -> Product/1
  Add1/1 -> Out/1

== system model_affc/Experiment & Haptics/Hypotrochoid trajectory for AFFC/CrossFade6 ==
  In1 : Inport
  In2 : Inport  Port=2
  AmountIn2 : Inport  Port=3
  Add : Sum  Inputs=+-
  Add1 : Sum
  One : Constant
  Product : Product  RndMeth=Zero
  Product1 : Product  RndMeth=Zero
  Saturation : Saturate  UpperLimit=1  LowerLimit=0
  Out : Outport
  wires:
  In1/1 -> Product1/1
  AmountIn2/1 -> Saturation/1
  One/1 -> Add/1
  Saturation/1 -> Product/2, Add/2
  Add/1 -> Product1/2
  Product/1 -> Add1/2
  Product1/1 -> Add1/1
  In2/1 -> Product/1
  Add1/1 -> Out/1

== system model_affc/Experiment & Haptics/Hypotrochoid trajectory for AFFC/Cycloid ==
  note: Given a linear input 0<=in<=1, it gives a cycloid output 0<=out<=1.
      | If In is outside the 0..1 range, it is limited to 0 or 1.
  In : Inport
  Gain1 : Gain  Gain=2*pi
  Gain2 : Gain  Gain=1/(2*pi)
  Saturation : Saturate  UpperLimit=1  LowerLimit=0
  Subtract : Sum  Inputs=+-
  Trigonometric Function : Trigonometry
  Out : Outport
  wires:
  Gain1/1 -> Trigonometric Function/1
  Subtract/1 -> Out/1
  In/1 -> Saturation/1
  Saturation/1 -> Gain1/1, Subtract/1
  Trigonometric Function/1 -> Gain2/1
  Gain2/1 -> Subtract/2

== system model_affc/Experiment & Haptics/Hypotrochoid trajectory for AFFC/Cycloid1 ==
  note: Given a linear input 0<=in<=1, it gives a cycloid output 0<=out<=1.
      | If In is outside the 0..1 range, it is limited to 0 or 1.
  In : Inport
  Gain1 : Gain  Gain=2*pi
  Gain2 : Gain  Gain=1/(2*pi)
  Saturation : Saturate  UpperLimit=1  LowerLimit=0
  Subtract : Sum  Inputs=+-
  Trigonometric Function : Trigonometry
  Out : Outport
  wires:
  Gain1/1 -> Trigonometric Function/1
  Subtract/1 -> Out/1
  In/1 -> Saturation/1
  Saturation/1 -> Gain1/1, Subtract/1
  Trigonometric Function/1 -> Gain2/1
  Gain2/1 -> Subtract/2

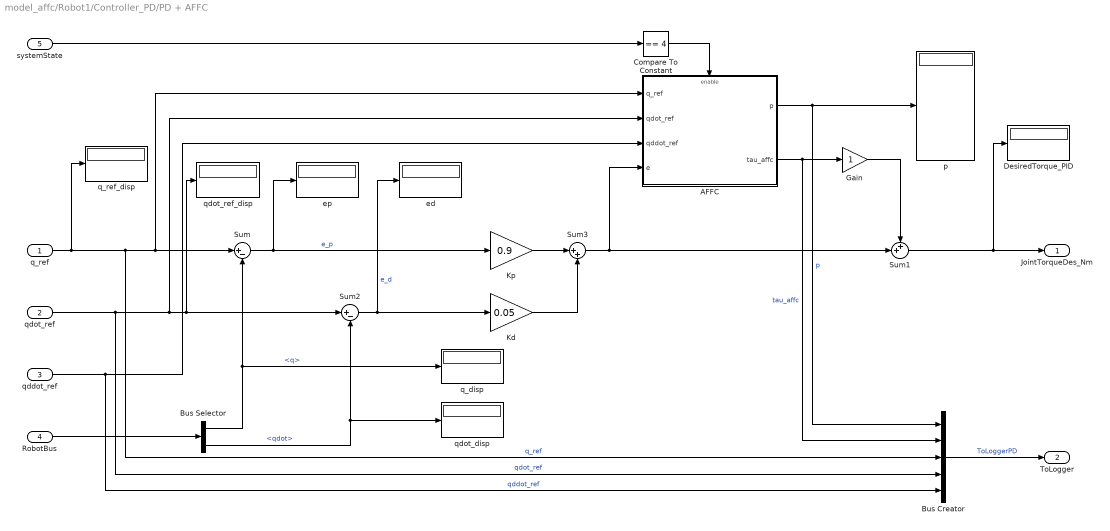
== system model_affc/Robot1/Controller_PD/PD + AFFC ==
  q_ref : Inport
  qdot_ref : Inport  Port=2
  qddot_ref : Inport  Port=3
  RobotBus : Inport  Port=4
  systemState : Inport  Port=5
  AFFC : Subsystem
  Bus Creator : BusCreator  Inputs=5
  Bus Selector : BusSelector  OutputSignals=qJointSpace.q,qJointSpace.qdot
  Compare To Constant : simulink/Logic and Bit Operations/Compare To Constant  relop===  const=4  OutDataTypeStr=boolean
  DesiredTorque_PID : Display
  Gain : Gain
  Kd : Gain  Gain=0.05
  Kp : Gain  Gain=0.9
  Sum : Sum  Inputs=|+-
  Sum1 : Sum  Inputs=++|
  Sum2 : Sum  Inputs=|+-
  Sum3 : Sum  Inputs=|++
  ed : Display
  ep : Display
  p : Display
  q_disp : Display
  q_ref_disp : Display
  qdot_disp : Display
  qdot_ref_disp : Display
  JointTorqueDes_Nm : Outport
  ToLogger : Outport  Port=2
  wires:
  Bus Creator/1 -> ToLogger/1  "ToLoggerPD"
  Compare To Constant/1 -> AFFC/Enable
  systemState/1 -> Compare To Constant/1
  AFFC/2(tau_affc) -> Gain/1, Bus Creator/2  "tau_affc"
  AFFC/1(p) -> p/1, Bus Creator/1  "p"
  qddot_ref/1 -> AFFC/3(qddot_ref), Bus Creator/5  "qddot_ref"
  RobotBus/1 -> Bus Selector/1
  Sum1/1 -> DesiredTorque_PID/1, JointTorqueDes_Nm/1
  Gain/1 -> Sum1/1
  Sum2/1 -> ed/1, Kd/1  "e_d"
  qdot_ref/1 -> qdot_ref_disp/1, Sum2/1, AFFC/2(qdot_ref), Bus Creator/4  "qdot_ref"
  Kp/1 -> Sum3/1
  Kd/1 -> Sum3/2
  Sum3/1 -> Sum1/2, AFFC/4(e)
  Sum/1 -> ep/1, Kp/1  "e_p"
  q_ref/1 -> q_ref_disp/1, Sum/1, AFFC/1(q_ref), Bus Creator/3  "q_ref"
  Bus Selector/1 -> q_disp/1, Sum/2  "<q>"
  Bus Selector/2 -> qdot_disp/1, Sum2/2  "<qdot>"

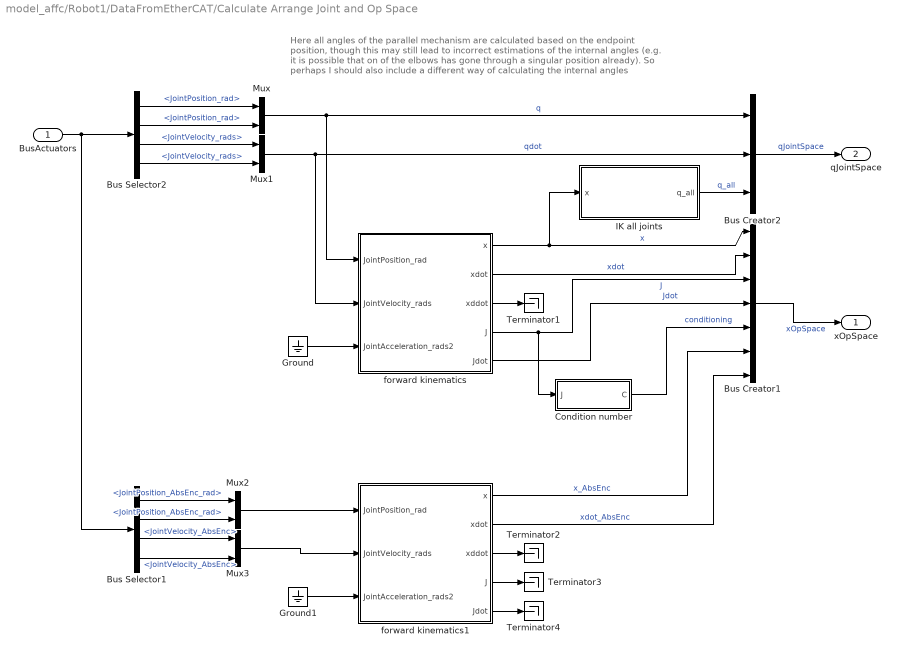
== system model_affc/Robot1/DataFromEtherCAT/Calculate Arrange Joint and Op Space ==
  note: Here all angles of the parallel mechanism are calculated
      | based on the endpoint position, though this may still lead to incorrect
      | estimations of the internal angles (e.g. it is possible that on of the elbows
      | has gone through a singular position already). So perhaps I should also include
      | a different way of calculating the internal angles
  BusActuators : Inport
  Bus Creator1 : BusCreator  Inputs=7
  Bus Creator2 : BusCreator  Inputs=3
  Bus Selector1 : BusSelector  OutputSignals=BusActuator1.JointPosition_AbsEnc_rad,BusActuator2.JointPosition_AbsEnc_rad,BusActuator1.JointVelocity_AbsEnc,BusActuator2.JointVelocity_AbsEnc
  Bus Selector2 : BusSelector  OutputSignals=BusActuator1.JointPosition_rad,BusActuator2.JointPosition_rad,BusActuator1.JointVelocity_rads,BusActuator2.JointVelocity_rads
  Condition number : MATLAB Function  TreatAsAtomicUnit=on
  Ground : Ground
  Ground1 : Ground
  IK all joints : MATLAB Function  TreatAsAtomicUnit=on
  Mux{,1..3} (4 alike) : Mux  Inputs=2
  Terminator{1..4} (4 alike) : Terminator
  forward kinematics : Subsystem
  forward kinematics1 : Subsystem
  xOpSpace : Outport
  qJointSpace : Outport  Port=2
  wires:
  forward kinematics/5(Jdot) -> Bus Creator1/4  "Jdot"
  forward kinematics/3(xddot) -> Terminator1/1
  forward kinematics/2(xdot) -> Bus Creator1/2  "xdot"
  forward kinematics/1(x) -> IK all joints/1(x), Bus Creator1/1  "x"
  Bus Creator1/1 -> xOpSpace/1  "xOpSpace"
  forward kinematics/4(J) -> Condition number/1(J), Bus Creator1/3  "J"
  Ground/1 -> forward kinematics/3(JointAcceleration_rads2)
  Bus Creator2/1 -> qJointSpace/1  "qJointSpace"
  BusActuators/1 -> Bus Selector1/1, Bus Selector2/1
  Bus Selector2/1 -> Mux/1  "<JointPosition_rad>"
  Bus Selector2/2 -> Mux/2  "<JointPosition_rad>"
  Bus Selector2/3 -> Mux1/1  "<JointVelocity_rads>"
  Bus Selector2/4 -> Mux1/2  "<JointVelocity_rads>"
  Mux1/1 -> forward kinematics/2(JointVelocity_rads), Bus Creator2/2  "qdot"
  Mux/1 -> forward kinematics/1(JointPosition_rad), Bus Creator2/1  "q"
  IK all joints/1(q_all) -> Bus Creator2/3  "q_all"
  Condition number/1(C) -> Bus Creator1/5  "conditioning"
  Bus Selector1/4 -> Mux3/2  "<JointVelocity_AbsEnc>"
  Bus Selector1/3 -> Mux3/1  "<JointVelocity_AbsEnc>"
  Bus Selector1/2 -> Mux2/2  "<JointPosition_AbsEnc_rad>"
  Bus Selector1/1 -> Mux2/1  "<JointPosition_AbsEnc_rad>"
  forward kinematics1/3(xddot) -> Terminator2/1
  Ground1/1 -> forward kinematics1/3(JointAcceleration_rads2)
  Mux2/1 -> forward kinematics1/1(JointPosition_rad)
  Mux3/1 -> forward kinematics1/2(JointVelocity_rads)
  forward kinematics1/2(xdot) -> Bus Creator1/7  "xdot_AbsEnc"
  forward kinematics1/1(x) -> Bus Creator1/6  "x_AbsEnc"
  forward kinematics1/4(J) -> Terminator3/1
  forward kinematics1/5(Jdot) -> Terminator4/1

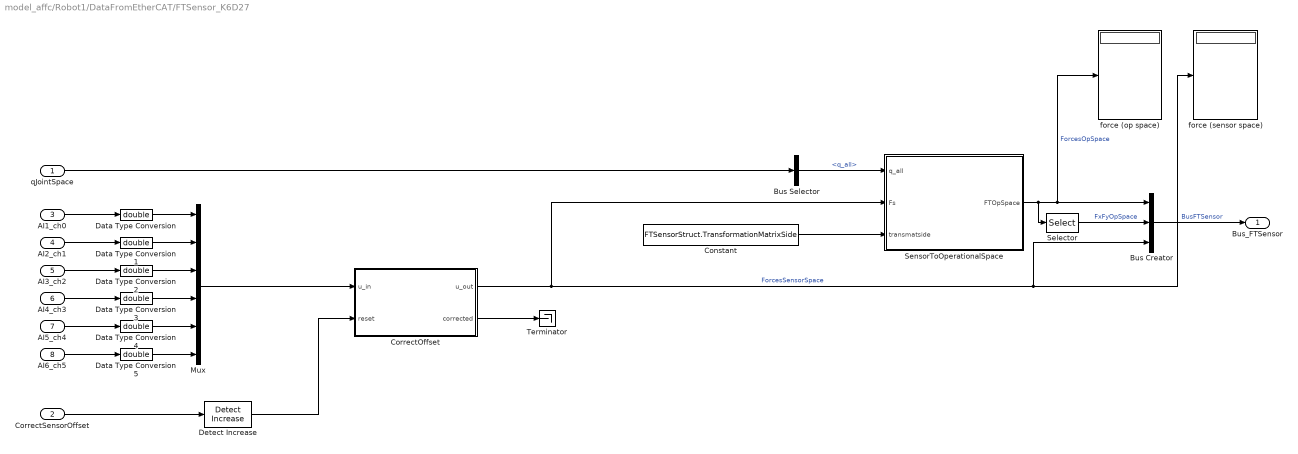
== system model_affc/Robot1/DataFromEtherCAT/FTSensor_K6D27 ==
  qJointSpace : Inport
  CorrectSensorOffset : Inport  Port=2
  AI1_ch0 : Inport  Port=3
  AI2_ch1 : Inport  Port=4
  AI3_ch2 : Inport  Port=5
  AI4_ch3 : Inport  Port=6
  AI5_ch4 : Inport  Port=7
  AI6_ch5 : Inport  Port=8
  Bus Creator : BusCreator  Inputs=3
  Bus Selector : BusSelector  OutputSignals=q_all
  Constant : Constant  Value=FTSensorStruct.TransformationMatrixSide
  CorrectOffset : MATLAB Function  TreatAsAtomicUnit=on
  Data Type Conversion{,1..5} (6 alike) : DataTypeConversion  OutDataTypeStr=double
  Detect Increase : simulink/Logic and Bit Operations/Detect Increase  vinit=0.0  InputProcessing=Inherited  OutDataTypeStr=boolean
  Mux : Mux  Inputs=6
  Selector : Selector  InputPortWidth=6  IndexOptions=Index vector (dialog)  Indices=[1 2]  OutputSizes=1
  SensorToOperationalSpace : MATLAB Function  TreatAsAtomicUnit=on
  Terminator : Terminator
  force (op space) : Display
  force (sensor space) : Display
  Bus_FTSensor : Outport
  wires:
  Constant/1 -> SensorToOperationalSpace/3(transmatside)
  Bus Creator/1 -> Bus_FTSensor/1  "BusFTSensor"
  SensorToOperationalSpace/1(FTOpSpace) -> Selector/1, force (op space)/1, Bus Creator/1  "ForcesOpSpace"
  Data Type Conversion5/1 -> Mux/6
  Data Type Conversion4/1 -> Mux/5
  Data Type Conversion3/1 -> Mux/4
  Data Type Conversion2/1 -> Mux/3
  Data Type Conversion1/1 -> Mux/2
  Data Type Conversion/1 -> Mux/1
  CorrectOffset/1(u_out) -> SensorToOperationalSpace/2(Fs), Bus Creator/3, force (sensor space)/1  "ForcesSensorSpace"
  CorrectOffset/2(corrected) -> Terminator/1
  AI3_ch2/1 -> Data Type Conversion2/1
  AI4_ch3/1 -> Data Type Conversion3/1
  AI5_ch4/1 -> Data Type Conversion4/1
  AI6_ch5/1 -> Data Type Conversion5/1
  Detect Increase/1 -> CorrectOffset/2(reset)
  CorrectSensorOffset/1 -> Detect Increase/1
  Mux/1 -> CorrectOffset/1(u_in)
  AI1_ch0/1 -> Data Type Conversion/1
  AI2_ch1/1 -> Data Type Conversion1/1
  qJointSpace/1 -> Bus Selector/1
  Bus Selector/1 -> SensorToOperationalSpace/1(q_all)  "<q_all>"
  Selector/1 -> Bus Creator/2  "FxFyOpSpace"

== system model_affc/Robot1/DataToEtherCAT/CreateSingleErrorValue1 ==
  ErrorChecks : Inport
  Data Type Conversion1 : DataTypeConversion  OutDataTypeStr=double
  ErrorToPower2 : MATLAB Function  TreatAsAtomicUnit=on
  ErrorValue : Outport
  wires:
  Data Type Conversion1/1 -> ErrorToPower2/1(u)
  ErrorChecks/1 -> Data Type Conversion1/1
  ErrorToPower2/1(e) -> ErrorValue/1

== system model_affc/Robot1/DataToEtherCAT/CreateSingleErrorValue2 ==
  ErrorChecks : Inport
  Data Type Conversion1 : DataTypeConversion  OutDataTypeStr=double
  ErrorToPower2 : MATLAB Function  TreatAsAtomicUnit=on
  ErrorValue : Outport
  wires:
  Data Type Conversion1/1 -> ErrorToPower2/1(u)
  ErrorChecks/1 -> Data Type Conversion1/1
  ErrorToPower2/1(e) -> ErrorValue/1

== system model_affc/Robot1/DataToEtherCAT/FTSensorError ==
  RobotBus : Inport
  AvoidAlgebraicLoop : Memory
  Bus Selector : BusSelector  OutputSignals=BusFTSensor.ForcesSensorSpace
  Constant : Constant  Value=RobotStruct.FTSensor.MaxAllowableForcesTorqueSensor
  Data Type Conversion1 : DataTypeConversion  OutDataTypeStr=boolean
  Detect Change : simulink/Logic and Bit Operations/Detect Change  vinit=0  InputProcessing=Inherited  OutDataTypeStr=boolean
  FTSensorLastError : Display
  LatchRising : LibraryFM/Utilities/LatchRising  ic=0
  MATLAB Function : MATLAB Function  TreatAsAtomicUnit=on
  ShowFTSensorErrorLatched : Display
  FTSensorError : Outport
  FTSensorErrorLatched : Outport  Port=2
  wires:
  Constant/1 -> MATLAB Function/2(MaxForcesTorques)
  MATLAB Function/1(e) -> Data Type Conversion1/1, FTSensorLastError/1
  LatchRising/1 -> ShowFTSensorErrorLatched/1, FTSensorErrorLatched/1
  AvoidAlgebraicLoop/1 -> Detect Change/1, LatchRising/1, FTSensorError/1
  Detect Change/1 -> LatchRising/Trigger
  RobotBus/1 -> Bus Selector/1
  Bus Selector/1 -> MATLAB Function/1(ForcesTorques)  "<ForcesSensorSpace>"
  Data Type Conversion1/1 -> AvoidAlgebraicLoop/1

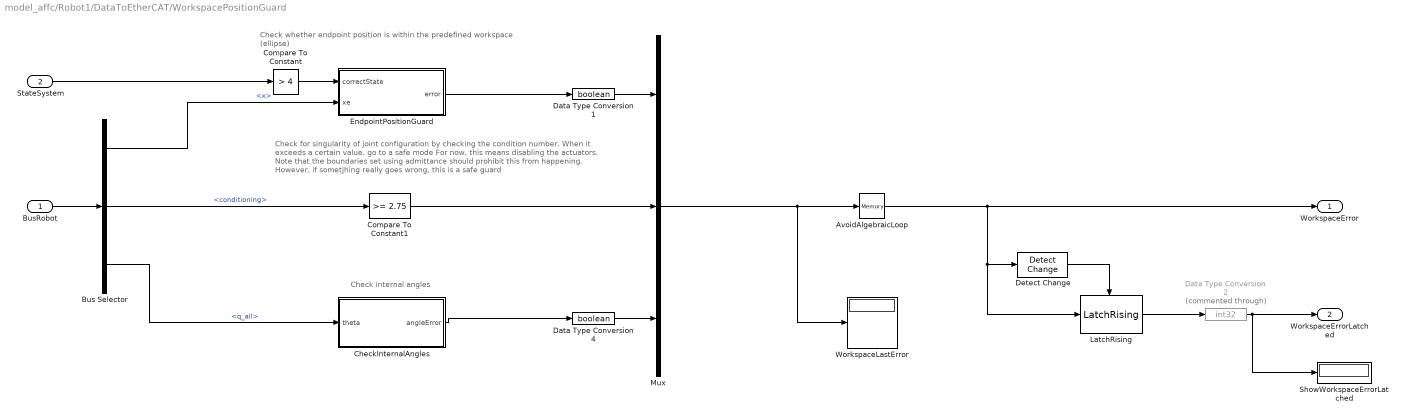
== system model_affc/Robot1/DataToEtherCAT/WorkspacePositionGuard ==
  note: Check internal angles
  note: Check whether endpoint position is within the predefined workspace
      | (ellipse)
  note: Check for singularity of joint configuration by checking
      | the condition number. When it exceeds a certain value, go to a safe mode
      | For now, this means disabling the actuators.
      | Note that the boundaries set using admittance should prohibit this from happening.
      | However, if sometjhing really goes wrong, this is a safe guard
  BusRobot : Inport
  StateSystem : Inport  Port=2
  AvoidAlgebraicLoop : Memory
  Bus Selector : BusSelector  OutputSignals=xOpSpace.x,xOpSpace.conditioning,qJointSpace.q_all
  CheckInternalAngles : MATLAB Function  TreatAsAtomicUnit=on
  Compare To Constant : simulink/Logic and Bit Operations/Compare To Constant  relop=>  const=4  OutDataTypeStr=boolean
  Compare To Constant1 : simulink/Logic and Bit Operations/Compare To Constant  relop=>=  const=2.75  OutDataTypeStr=boolean
  Data Type Conversion1 : DataTypeConversion  OutDataTypeStr=boolean
  Data Type Conversion2 : DataTypeConversion  Commented=through  OutDataTypeStr=int32
  Data Type Conversion4 : DataTypeConversion  OutDataTypeStr=boolean
  Detect Change : simulink/Logic and Bit Operations/Detect Change  vinit=0  InputProcessing=Inherited  OutDataTypeStr=boolean
  EndpointPositionGuard : MATLAB Function  TreatAsAtomicUnit=on
  LatchRising : LibraryFM/Utilities/LatchRising  ic=0
  Mux : Mux  Inputs=3
  ShowWorkspaceErrorLatched : Display
  WorkspaceLastError : Display
  WorkspaceError : Outport
  WorkspaceErrorLatched : Outport  Port=2
  wires:
  BusRobot/1 -> Bus Selector/1
  Bus Selector/1 -> EndpointPositionGuard/2(xe)  "<x>"
  LatchRising/1 -> Data Type Conversion2/1
  EndpointPositionGuard/1(error) -> Data Type Conversion1/1
  Mux/1 -> AvoidAlgebraicLoop/1, WorkspaceLastError/1
  Detect Change/1 -> LatchRising/Trigger
  AvoidAlgebraicLoop/1 -> WorkspaceError/1, Detect Change/1, LatchRising/1
  Compare To Constant/1 -> EndpointPositionGuard/1(correctState)
  Bus Selector/2 -> Compare To Constant1/1  "<conditioning>"
  StateSystem/1 -> Compare To Constant/1
  Data Type Conversion2/1 -> WorkspaceErrorLatched/1, ShowWorkspaceErrorLatched/1
  Data Type Conversion1/1 -> Mux/1
  Compare To Constant1/1 -> Mux/2
  CheckInternalAngles/1(angleError) -> Data Type Conversion4/1
  Bus Selector/3 -> CheckInternalAngles/1(theta)  "<q_all>"
  Data Type Conversion4/1 -> Mux/3

== system model_affc/Robot1/Controller_PD/PD + AFFC/AFFC ==
  q_ref : Inport
  qdot_ref : Inport  Port=2
  qddot_ref : Inport  Port=3
  e : Inport  Port=4
  Enable : EnablePort  StatesWhenEnabling=reset
  AFFC : MATLAB Function  TreatAsAtomicUnit=on
  Counter Free-Running : simulink/Sources/Counter Free-Running  NumBits=32  tsamp=-1
  Data Type Conversion : DataTypeConversion  OutDataTypeStr=double
  Learning factors : Constant  Value=[1e-5;5e-3;5e-4;1e-3]
  sample time : Gain  Gain=sampleTime
  p : Outport  OutputWhenDisabled=reset  InitialOutput=zeros(7,1)
  tau_affc : Outport  Port=2  OutputWhenDisabled=reset  InitialOutput=[0;0]
  wires:
  e/1 -> AFFC/5(e)
  qddot_ref/1 -> AFFC/4(qddot)
  qdot_ref/1 -> AFFC/3(qdot)
  q_ref/1 -> AFFC/2(q)
  AFFC/2(tau) -> tau_affc/1
  AFFC/1(p) -> p/1
  Counter Free-Running/1 -> Data Type Conversion/1
  sample time/1 -> AFFC/1(t)
  Data Type Conversion/1 -> sample time/1
  Learning factors/1 -> AFFC/6(w)

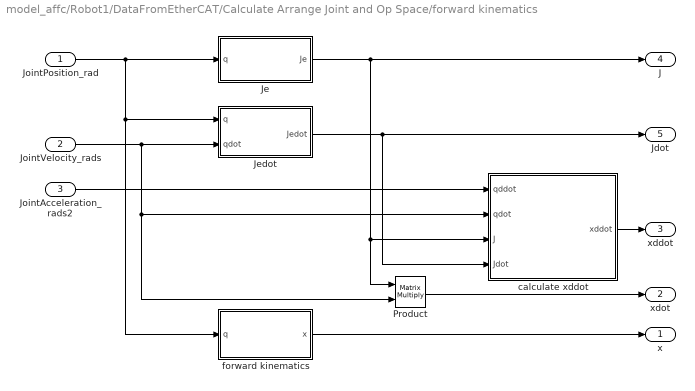
== system model_affc/Robot1/DataFromEtherCAT/Calculate Arrange Joint and Op Space/forward kinematics ==
  JointPosition_rad : Inport  PortDimensions=[2 1]
  JointVelocity_rads : Inport  Port=2  PortDimensions=[2 1]
  JointAcceleration_rads2 : Inport  Port=3  PortDimensions=[2 1]
  Je : MATLAB Function  TreatAsAtomicUnit=on
  Jedot : MATLAB Function  TreatAsAtomicUnit=on
  Product : Product  Multiplication=Matrix(*)
  calculate xddot : MATLAB Function  TreatAsAtomicUnit=on
  forward kinematics : MATLAB Function  TreatAsAtomicUnit=on
  x : Outport
  xdot : Outport  Port=2
  xddot : Outport  Port=3
  J : Outport  Port=4
  Jdot : Outport  Port=5
  wires:
  JointPosition_rad/1 -> forward kinematics/1(q), Jedot/1(q), Je/1(q)
  Je/1(Je) -> calculate xddot/3(J), Product/1, J/1
  JointVelocity_rads/1 -> calculate xddot/2(qdot), Product/2, Jedot/2(qdot)
  Jedot/1(Jedot) -> calculate xddot/4(Jdot), Jdot/1
  Product/1 -> xdot/1
  forward kinematics/1(x) -> x/1
  calculate xddot/1(xddot) -> xddot/1
  JointAcceleration_rads2/1 -> calculate xddot/1(qddot)

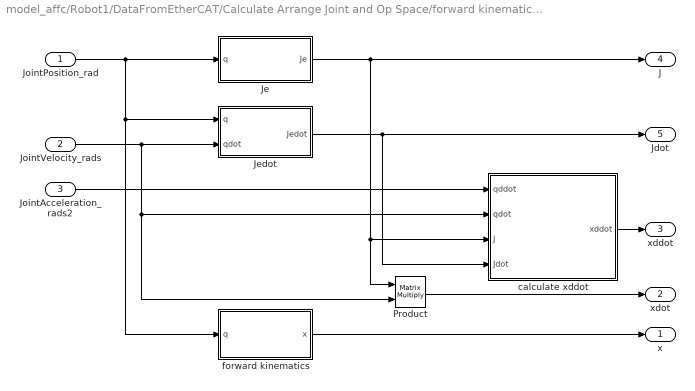
== system model_affc/Robot1/DataFromEtherCAT/Calculate Arrange Joint and Op Space/forward kinematics1 ==
  JointPosition_rad : Inport  PortDimensions=[2 1]
  JointVelocity_rads : Inport  Port=2  PortDimensions=[2 1]
  JointAcceleration_rads2 : Inport  Port=3  PortDimensions=[2 1]
  Je : MATLAB Function  TreatAsAtomicUnit=on
  Jedot : MATLAB Function  TreatAsAtomicUnit=on
  Product : Product  Multiplication=Matrix(*)
  calculate xddot : MATLAB Function  TreatAsAtomicUnit=on
  forward kinematics : MATLAB Function  TreatAsAtomicUnit=on
  x : Outport
  xdot : Outport  Port=2
  xddot : Outport  Port=3
  J : Outport  Port=4
  Jdot : Outport  Port=5
  wires:
  JointPosition_rad/1 -> forward kinematics/1(q), Jedot/1(q), Je/1(q)
  Je/1(Je) -> calculate xddot/3(J), Product/1, J/1
  JointVelocity_rads/1 -> calculate xddot/2(qdot), Product/2, Jedot/2(qdot)
  Jedot/1(Jedot) -> calculate xddot/4(Jdot), Jdot/1
  Product/1 -> xdot/1
  forward kinematics/1(x) -> x/1
  calculate xddot/1(xddot) -> xddot/1
  JointAcceleration_rads2/1 -> calculate xddot/1(qddot)

== matlab function model_affc/Experiment & Haptics/Hypotrochoid trajectory for AFFC/hypotrochoidal trajectory ==
  data: t input; p output; v output; a output; T input; n input; hstart input; hend input; wstart input; wend input
function [p,v,a] = fcn(t,T,n,hstart,hend,wstart,wend)
%#codegen

p = func_p_hypothrochoid(t,T,n,hstart,hend,wstart,wend);
v = func_v_hypothrochoid(t,T,n,hstart,hend,wstart,wend);
a = func_a_hypothrochoid(t,T,n,hstart,hend,wstart,wend);

== matlab function model_affc/Robot1/DataFromEtherCAT/Calculate Arrange Joint and Op Space/Condition number ==
  data: J input; C output
function C = conditioning(J)
%#codegen

C = norm(J)*norm(pinv(J));

== matlab function model_affc/Robot1/DataFromEtherCAT/Calculate Arrange Joint and Op Space/forward kinematics1/Je ==
  data: q input; Je output size=[2 2]; Lf parameter; Lu parameter; Lb parameter
function Je = Je( q, Lf, Lu, Lb)
%#codegen

% Calculate the Jacobian for this particular device configuration.
% Note that the function func_eq_Je needs to be in the libraries/kinematis_functions folder

% jacobians
Je = func_eq_Je(q(1),q(2),Lf,Lu,Lb);

== matlab function model_affc/Robot1/DataFromEtherCAT/Calculate Arrange Joint and Op Space/forward kinematics1/Jedot ==
  data: q input; qdot input; Jedot output size=[2 2]; Lf parameter; Lu parameter; Lb parameter
function Jedot = Jedot( q, qdot, Lf, Lu, Lb)
%#codegen

% Calculate the time derivative of the Jacobian for this particular device configuration.
% Note that the function func_eq_Je needs to be in the libraries/kinematis_functions folder


% jacobians
Jedot = func_eq_Jedot(q(1),q(2),qdot(1),qdot(2),Lf,Lu,Lb);

== matlab function model_affc/Robot1/DataFromEtherCAT/Calculate Arrange Joint and Op Space/forward kinematics1/calculate xddot ==
  data: qddot input; qdot input size=[2 1]; J input; xddot output size=[2 1]; Jdot input
function xddot = calc_xddot(qddot, qdot, J, Jdot)
%#codegen

xddot = J*qddot + Jdot*qdot;

== matlab function model_affc/Robot1/DataFromEtherCAT/Calculate Arrange Joint and Op Space/forward kinematics/forward kinematics ==
  data: q input; x output size=[2 1]; Lf parameter; Lu parameter; Lb parameter
function x = FK(q, Lf, Lu, Lb)
%#codegen

% Calculate the endpoint position (forward kinematics)
% Note that the function func_eq_FK needs to be in the libraries/kinematis_functions folder


x = func_eq_FK(q(1),q(2),Lf,Lu,Lb);

== matlab function model_affc/Robot1/DataFromEtherCAT/Calculate Arrange Joint and Op Space/forward kinematics1/forward kinematics ==
  data: q input; x output size=[2 1]; Lf parameter; Lu parameter; Lb parameter
function x = FK(q, Lf, Lu, Lb)
%#codegen

% Calculate the endpoint position (forward kinematics)
% Note that the function func_eq_FK needs to be in the libraries/kinematis_functions folder


x = func_eq_FK(q(1),q(2),Lf,Lu,Lb);
